simulink model "mediumFidelityScooterModel"  (R2022a)
settings: Solver=FixedStepAuto  StartTime=0  StopTime=50  FixedStep=Ts_mf  RelTol=1e-3  EnableMultiTasking=on
undefined symbols (not defined in the file): A, Cd, Crr, D, DiscIntNeverNeededParam, eff_gear, g, Ke, Kf, Ki_i, Ki_w, Kp_i, Kp_w, Kt, La, m_total, n_gear, Ra, rho, Rwheel, sigbuilder_block, slope, Tpeak, Vbat, Vnom
libraries: simulink x2, slpidlib x2
Description:
  | Medium fidelity simulation for control design validation
settings Model: Creator=The MathWorks, Inc.  LastModifiedBy=jdelolmo
settings SolverCC: AlgebraicLoopSolver=TrustRegion  AutoInsertRateTranBlk=on
settings DataIOCC: LimitDataPoints=on  ReturnWorkspaceOutputs=off
settings OptimizationCC: LifeSpan=inf
settings DebuggingCC: UnconnectedInputMsg=warning  UnconnectedOutputMsg=warning  UnconnectedLineMsg=warning  AllowSymbolicDim=off  SFUnexpectedBacktrackingDiag=warning  SFNoUnconditionalDefaultTransitionDiag=warning  SFExecutionAtInitializationDiag=none  SFMachineParentedDataDiag=warning  ArithmeticOperatorsInVariantConditions=warning
settings ModelReferenceCC: PropagateSignalLabelsOutOfModel=off
settings SFSimCC: SimUseLocalCustomCode=off  CustomCodeUndefinedFunction=UseInterfaceOnly
settings RTWCC: RTWUseLocalCustomCode=off  DLArmComputeVersion=19.05
settings CodeAppCC: StateflowObjectComments=on
settings GRTTargetCC: TargetLangStandard=C89/C90 (ANSI)
settings ConfigComp: CovMetricSettings=dw  CovSaveCumulativeToWorkspaceVar=on  CovSaveSingleToWorkspaceVar=on  CovExternalEMLEnable=off

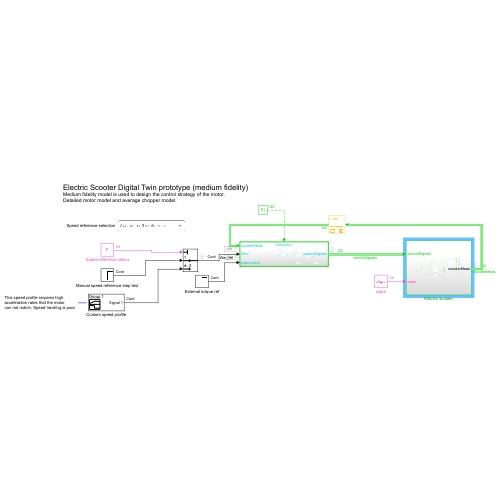
[thumbnail: Simulink's stored preview of the top-level diagram]
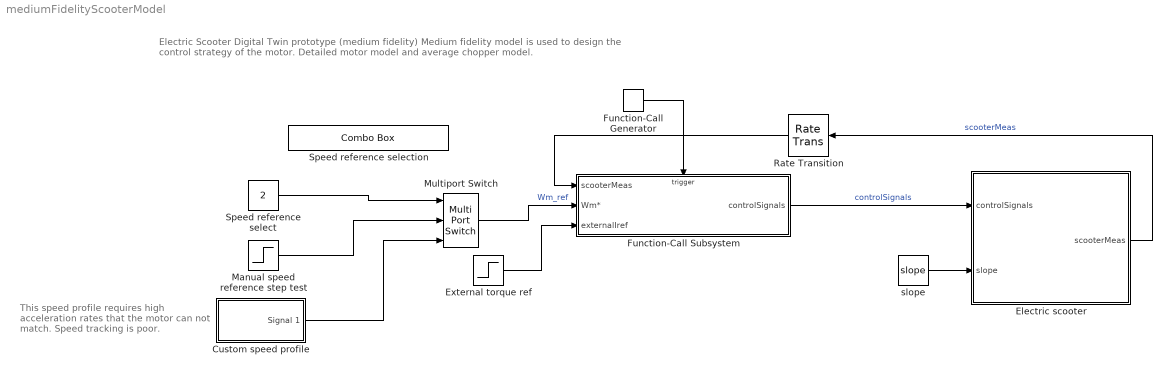
== system mediumFidelityScooterModel ==
  note: This speed profile requires high
      | acceleration rates that the motor
      | can not match. Speed tracking is poor.
  note: Electric Scooter Digital Twin prototype (medium fidelity)
      | Medium fidelity model is used to design the control strategy of the motor.
      | Detailed motor model and average chopper model.
  Custom speed profile : Subsystem  Tag=STV Subsys  LoadFcn=sigbuilder_block('load');  StartFcn=sigbuilder_block('start');  StopFcn=sigbuilder_block('stop');  ClipboardFcn=sigbuilder_block('clipboard');  mask(Sigbuilder block){tuvar=[0:10]}
      mask help: Simulink:masks:SigbuilderBlock_MD
      mask init:
      | if ~strcmp(get_param(bdroot(gcbh),'SimulationStatus'),'stopped') tuvar = sigbuilder_block('maskInit'); end
      settings: CopyFcn=sigbuilder_block('copy');  DeleteFcn=sigbuilder_block('delete');  ModelCloseFcn=sigbuilder_block('modelClose');  PreSaveFcn=sigbuilder_block('preSave');  PauseFcn=sigbuilder_block('pause');  ContinueFcn=sigbuilder_block('continue');  NameChangeFcn=sigbuilder_block('namechange');  OpenFcn=sigbuilder_block('open',[437.6 199.2 550.4 400 ]);  CloseFcn=sigbuilder_block('close');
      mask Display: plot(0, 0, 100, 100,[2, 2, 32, 32, 2], [68, 8, 8, 68, 68],[32, 2], [38, 38], [32, 19, 2],[53, 60, 44], [32, 17, 17, 2],[16, 16, 31, 31]);txt = getActiveGroup(gcbh);text(2, 100, txt,'verticalAlignment', 'top');
  Electric scooter : Subsystem
  External torque ref : Step  Time=0.1  After=Kt*16  SampleTime=0
  Function-Call Generator : simulink/Ports & Subsystems/Function-Call Generator  sample_time=Tcontrol  numberOfIterations=1  DisallowWideOutput=off
  Function-Call Subsystem : Subsystem  TreatAsAtomicUnit=on
  Manual speed reference step test : Step  Time=0.1  After=100  SampleTime=0
  Multiport Switch : MultiPortSwitch  Inputs=2  SaturateOnIntegerOverflow=off  InputSameDT=off
  Rate Transition : RateTransition  OutPortSampleTime=Tcontrol
  Speed reference select : Constant  Value=2
  Speed reference selection : ComboBox  LabelPosition=Hide  SelectedLabel=Custom profile reference
      settings: Values={{'Step reference', 'Custom profile reference', 'Vehicle profile'}, [1 2 3]}
  slope : Constant  Value=slope
  wires:
  Manual speed reference step test/1 -> Multiport Switch/2
  Speed reference select/1 -> Multiport Switch/1
  Custom speed profile/1(Signal 1) -> Multiport Switch/3
  slope/1 -> Electric scooter/2(slope)
  Function-Call Subsystem/1(controlSignals) -> Electric scooter/1(controlSignals)  "controlSignals"
  Function-Call Generator/1 -> Function-Call Subsystem/Trigger
  Electric scooter/1(scooterMeas) -> Rate Transition/1  "scooterMeas"
  Multiport Switch/1 -> Function-Call Subsystem/2(Wm*)  "Wm_ref"
  External torque ref/1 -> Function-Call Subsystem/3(externalIref)
  Rate Transition/1 -> Function-Call Subsystem/1(scooterMeas)

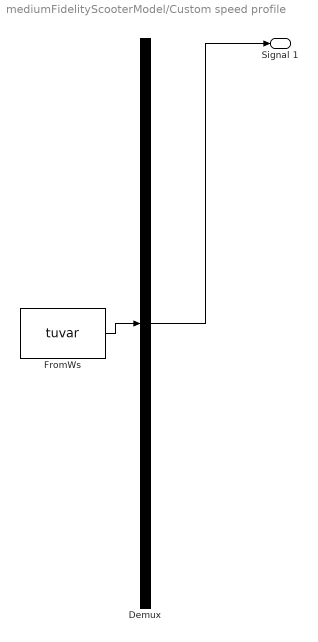
== system mediumFidelityScooterModel/Custom speed profile ==
  Demux : Demux  Tag=STV Demux  Outputs=1
      settings: DisplayOption=none
  FromWs : FromWorkspace  Tag=STV FromWs  VariableName=tuvar
      SigBuilderData=|
      | common.afterFinalStr = 'Extrapolate'
      | common.sampleTime = 0
      | dataSet.timeRange = [0 10]
      | dataSet.name = 'Group 1'
      | sbobj.Groups.Name = 'Group 1'
      | sbobj.Groups.Signals.Name = 'Signal 1'
      | sbobj.Groups.Signals.XData = [0 0.1 1.5 2 3 10]
      | sbobj.Groups.Signals.YData = [0 0 500 500 250 250]
  Signal 1 : Outport  Tag=STV Outport
  wires:
  Demux/1 -> Signal 1/1
  FromWs/1 -> Demux/1

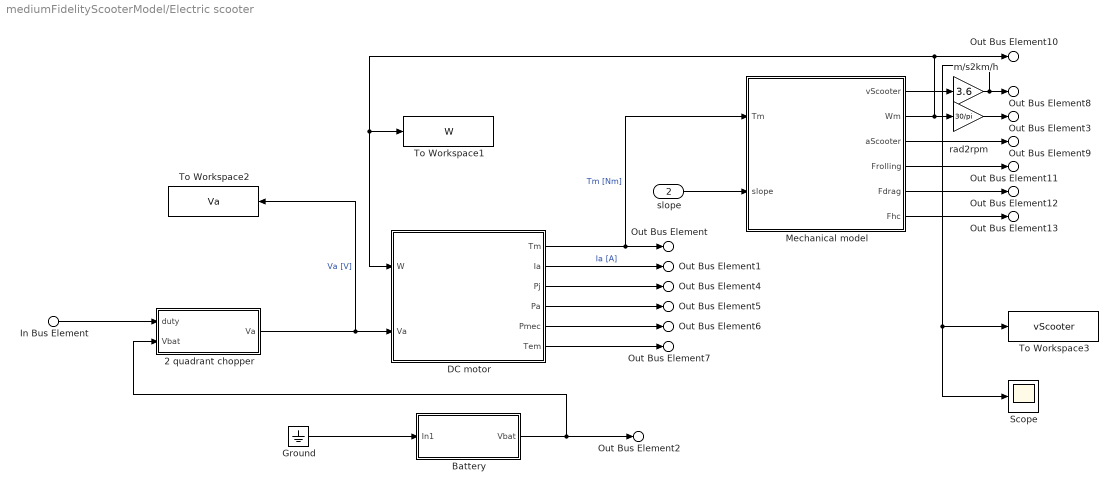
== system mediumFidelityScooterModel/Electric scooter ==
  In Bus Element : Inport  PortName=controlSignals  Element=duty
  slope : Inport  Port=2
  2 quadrant chopper : Subsystem
  Battery : Subsystem
  DC motor : Subsystem
  Ground : Ground
  Mechanical model : Subsystem
  Scope : Scope
  To Workspace1 : ToWorkspace  VariableName=W  SaveFormat=Timeseries  SampleTime=-1
  To Workspace2 : ToWorkspace  VariableName=Va  SaveFormat=Timeseries  SampleTime=-1
  To Workspace3 : ToWorkspace  VariableName=vScooter  SaveFormat=Timeseries  SampleTime=-1
  m/s2km/h : Gain  Gain=3.6
  rad2rpm : Gain  Gain=30/pi
  Out Bus Element : Outport  PortName=scooterMeas  Element=Tm
  Out Bus Element1 : Outport  PortName=scooterMeas  Element=Ia
  Out Bus Element2 : Outport  PortName=scooterMeas  Element=Vbat
  Out Bus Element4 : Outport  PortName=scooterMeas  Element=Pj
  Out Bus Element5 : Outport  PortName=scooterMeas  Element=Pa
  Out Bus Element6 : Outport  PortName=scooterMeas  Element=Pmec
  Out Bus Element7 : Outport  PortName=scooterMeas  Element=Tem
  Out Bus Element3 : Outport  PortName=scooterMeas  Element=WmRPM
  Out Bus Element8 : Outport  PortName=scooterMeas  Element=vScooter
  Out Bus Element9 : Outport  PortName=scooterMeas  Element=aScooter
  Out Bus Element10 : Outport  PortName=scooterMeas  Element=Wm
  Out Bus Element11 : Outport  PortName=scooterMeas  Element=Frolling
  Out Bus Element12 : Outport  PortName=scooterMeas  Element=Fdrag
  Out Bus Element13 : Outport  PortName=scooterMeas  Element=Fhc
  wires:
  DC motor/1(Tm) -> Mechanical model/1(Tm), Out Bus Element/1  "Tm [Nm]"
  DC motor/2(Ia) -> Out Bus Element1/1  "Ia [A]"
  Battery/1(Vbat) -> Out Bus Element2/1, 2 quadrant chopper/2(Vbat)
  Ground/1 -> Battery/1(In1)
  In Bus Element/1 -> 2 quadrant chopper/1(duty)
  2 quadrant chopper/1(Va) -> To Workspace2/1, DC motor/2(Va)  "Va [V]"
  DC motor/3(Pj) -> Out Bus Element4/1
  DC motor/4(Pa) -> Out Bus Element5/1
  DC motor/5(Pmec) -> Out Bus Element6/1
  DC motor/6(Tem) -> Out Bus Element7/1
  rad2rpm/1 -> Out Bus Element3/1
  Mechanical model/1(vScooter) -> m/s2km/h/1
  Mechanical model/2(Wm) -> rad2rpm/1, Out Bus Element10/1, To Workspace1/1, DC motor/1(W)
  Mechanical model/3(aScooter) -> Out Bus Element9/1
  slope/1 -> Mechanical model/2(slope)
  Mechanical model/4(Frolling) -> Out Bus Element11/1
  Mechanical model/5(Fdrag) -> Out Bus Element12/1
  Mechanical model/6(Fhc) -> Out Bus Element13/1
  m/s2km/h/1 -> Scope/1, To Workspace3/1, Out Bus Element8/1

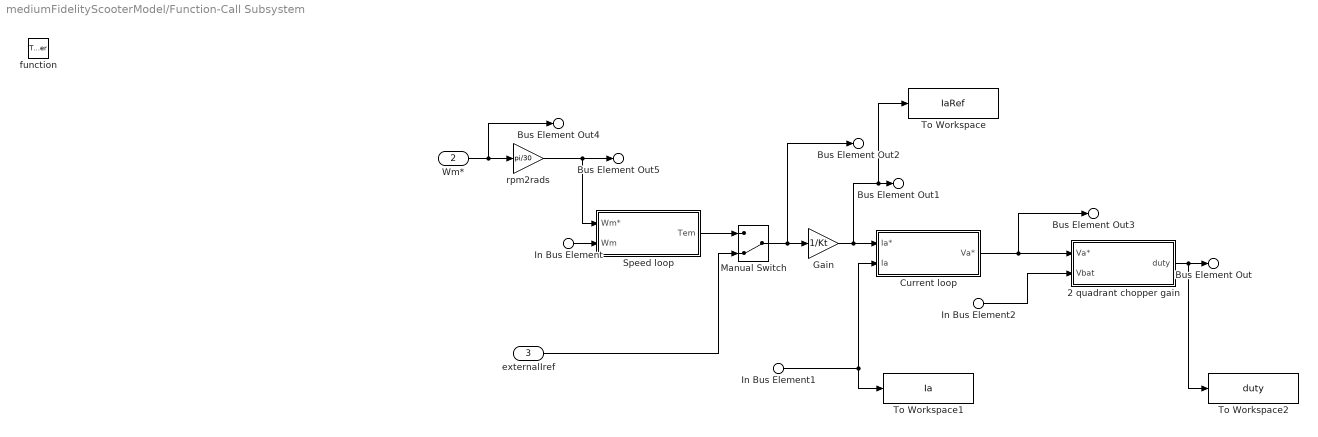
== system mediumFidelityScooterModel/Function-Call Subsystem ==
  In Bus Element1 : Inport  PortName=scooterMeas  Element=Ia
  In Bus Element : Inport  PortName=scooterMeas  Element=Wm
  In Bus Element2 : Inport  PortName=scooterMeas  Element=Vbat
  Wm* : Inport  Port=2
  externalIref : Inport  Port=3
  function : TriggerPort  TriggerType=function-call  VariantControl=(inherit)
  2 quadrant chopper gain : Subsystem
  Current loop : Subsystem
  Gain : Gain  Gain=1/Kt
  Manual Switch : ManualSwitch  CurrentSetting=0
  Speed loop : Subsystem
  To Workspace : ToWorkspace  VariableName=IaRef  SaveFormat=Timeseries  SampleTime=-1
  To Workspace1 : ToWorkspace  VariableName=Ia  SaveFormat=Timeseries  SampleTime=-1
  To Workspace2 : ToWorkspace  VariableName=duty  SaveFormat=Timeseries  SampleTime=-1
  rpm2rads : Gain  Gain=pi/30
  Bus Element Out : Outport  PortName=controlSignals  Element=duty
  Bus Element Out1 : Outport  PortName=controlSignals  Element=IaRef
  Bus Element Out2 : Outport  PortName=controlSignals  Element=TemRef
  Bus Element Out3 : Outport  PortName=controlSignals  Element=VaRef
  Bus Element Out4 : Outport  PortName=controlSignals  Element=WmRefRpm
  Bus Element Out5 : Outport  PortName=controlSignals  Element=WmRefRadS
  wires:
  externalIref/1 -> Manual Switch/2
  Wm*/1 -> Bus Element Out4/1, rpm2rads/1
  rpm2rads/1 -> Bus Element Out5/1, Speed loop/1(Wm*)
  Gain/1 -> To Workspace/1, Bus Element Out1/1, Current loop/1(Ia*)
  Speed loop/1(Tem) -> Manual Switch/1
  2 quadrant chopper gain/1(duty) -> To Workspace2/1, Bus Element Out/1
  In Bus Element/1 -> Speed loop/2(Wm)
  In Bus Element1/1 -> To Workspace1/1, Current loop/2(Ia)
  In Bus Element2/1 -> 2 quadrant chopper gain/2(Vbat)
  Current loop/1(Va*) -> Bus Element Out3/1, 2 quadrant chopper gain/1(Va*)
  Manual Switch/1 -> Bus Element Out2/1, Gain/1

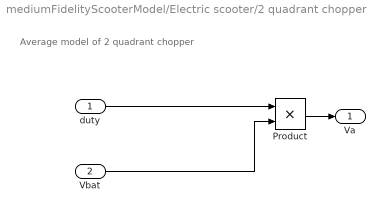
== system mediumFidelityScooterModel/Electric scooter/2 quadrant chopper ==
  note: Average model of 2 quadrant chopper
  duty : Inport
  Vbat : Inport  Port=2
  Product : Product
  Va : Outport
  wires:
  Vbat/1 -> Product/2
  duty/1 -> Product/1
  Product/1 -> Va/1

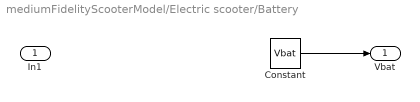
== system mediumFidelityScooterModel/Electric scooter/Battery ==
  In1 : Inport
  Constant : Constant  Value=Vbat
  Vbat : Outport
  wires:
  Constant/1 -> Vbat/1

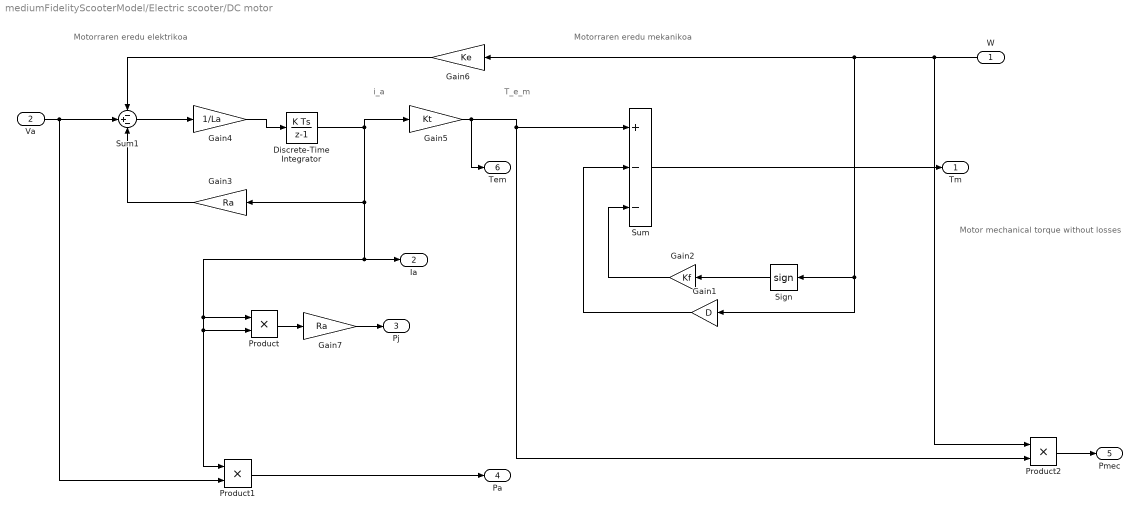
== system mediumFidelityScooterModel/Electric scooter/DC motor ==
  note: Motor mechanical torque without losses
  note: Motorraren eredu mekanikoa
  note: T_e_m
  note: Motorraren eredu elektrikoa
  note: i_a
  W : Inport
  Va : Inport  Port=2
  Discrete-Time Integrator : DiscreteIntegrator  SampleTime=200e-6  ICPrevOutput=DiscIntNeverNeededParam  ICPrevScaledInput=DiscIntNeverNeededParam
  Gain1 : Gain  Gain=D
  Gain2 : Gain  Gain=Kf
  Gain3 : Gain  Gain=Ra
  Gain4 : Gain  Gain=1/La
  Gain5 : Gain  Gain=Kt
  Gain6 : Gain  Gain=Ke
  Gain7 : Gain  Gain=Ra
  Product : Product
  Product1 : Product
  Product2 : Product
  Sign : Signum
  Sum : Sum  Inputs=+--
  Sum1 : Sum  Inputs=-+-
  Tm : Outport  VectorParamsAs1DForOutWhenUnconnected=off
  Ia : Outport  Port=2  VectorParamsAs1DForOutWhenUnconnected=off
  Pj : Outport  Port=3  VectorParamsAs1DForOutWhenUnconnected=off
  Pa : Outport  Port=4  VectorParamsAs1DForOutWhenUnconnected=off
  Pmec : Outport  Port=5  VectorParamsAs1DForOutWhenUnconnected=off
  Tem : Outport  Port=6  VectorParamsAs1DForOutWhenUnconnected=off
  wires:
  Gain4/1 -> Discrete-Time Integrator/1
  Sum1/1 -> Gain4/1
  Sign/1 -> Gain2/1
  Gain3/1 -> Sum1/3
  Gain1/1 -> Sum/2
  Va/1 -> Product1/2, Sum1/2
  Gain5/1 -> Tem/1, Sum/1, Product2/2
  Sum/1 -> Tm/1
  Discrete-Time Integrator/1 -> Gain5/1, Product/1, Product/2, Product1/1, Ia/1, Gain3/1
  Gain6/1 -> Sum1/1
  Gain7/1 -> Pj/1
  Product/1 -> Gain7/1
  Product1/1 -> Pa/1
  Product2/1 -> Pmec/1
  Gain2/1 -> Sum/3
  W/1 -> Product2/1, Gain1/1, Sign/1, Gain6/1

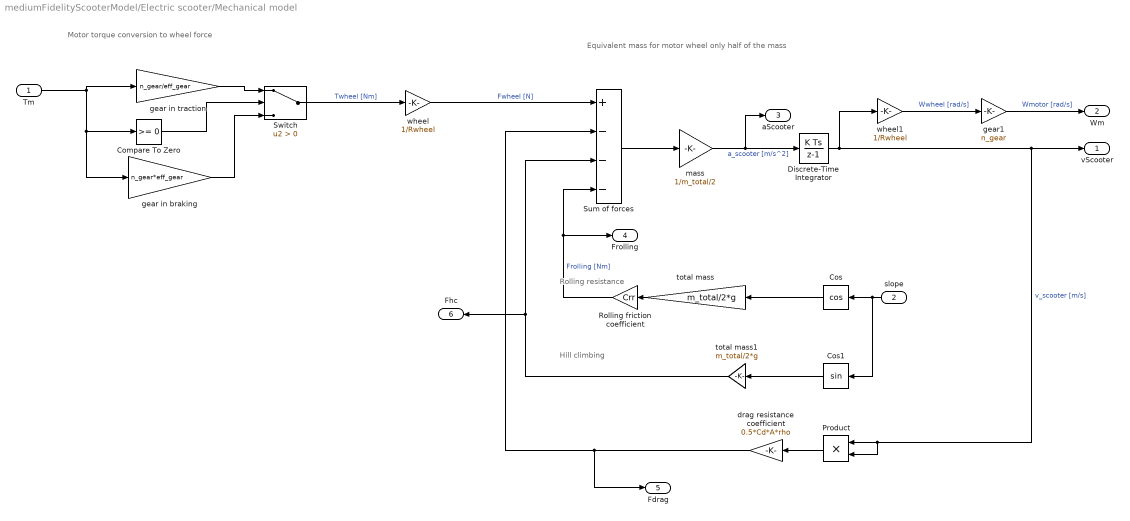
== system mediumFidelityScooterModel/Electric scooter/Mechanical model ==
  note: Hill climbing
  note: Motor torque conversion to wheel force
  note: Equivalent mass for motor wheel only half of the mass
  note: Rolling resistance
  Tm : Inport
  slope : Inport  Port=2
  Compare To Zero : simulink/Logic and Bit Operations/Compare To Zero  relop=>=  OutDataTypeStr=boolean
  Cos : Trigonometry  Operator=cos
  Cos1 : Trigonometry
  Discrete-Time Integrator : DiscreteIntegrator  SampleTime=200e-6  ICPrevOutput=DiscIntNeverNeededParam  ICPrevScaledInput=DiscIntNeverNeededParam
  Product : Product
  Rolling friction coefficient : Gain  Gain=Crr
  Sum of forces : Sum  Inputs=+---
  Switch : Switch  Criteria=u2 > Threshold  SaturateOnIntegerOverflow=off  InputSameDT=off
  drag resistance coefficient : Gain  Gain=0.5*Cd*A*rho
  gear in braking : Gain  Gain=n_gear*eff_gear
  gear in traction : Gain  Gain=n_gear/eff_gear
  gear1 : Gain  Gain=n_gear
  mass : Gain  Gain=1/m_total/2
  total mass : Gain  Gain=m_total/2*g
  total mass1 : Gain  Gain=m_total/2*g
  wheel : Gain  Gain=1/Rwheel
  wheel1 : Gain  Gain=1/Rwheel
  vScooter : Outport
  Wm : Outport  Port=2
  aScooter : Outport  Port=3
  Frolling : Outport  Port=4
  Fdrag : Outport  Port=5
  Fhc : Outport  Port=6
  wires:
  Tm/1 -> Compare To Zero/1, gear in braking/1, gear in traction/1
  wheel/1 -> Sum of forces/1  "Fwheel [N]"
  Sum of forces/1 -> mass/1
  mass/1 -> Discrete-Time Integrator/1, aScooter/1  "a_scooter [m/s^2]"
  Discrete-Time Integrator/1 -> Product/2, Product/1, vScooter/1, wheel1/1  "v_scooter [m/s]"
  wheel1/1 -> gear1/1  "Wwheel [rad/s]"
  gear1/1 -> Wm/1  "Wmotor [rad/s]"
  Switch/1 -> wheel/1  "Twheel [Nm]"
  gear in traction/1 -> Switch/1
  gear in braking/1 -> Switch/3
  Compare To Zero/1 -> Switch/2
  Rolling friction coefficient/1 -> Frolling/1, Sum of forces/4  "Frolling [Nm]"
  total mass/1 -> Rolling friction coefficient/1
  Cos/1 -> total mass/1
  slope/1 -> Cos1/1, Cos/1
  Cos1/1 -> total mass1/1
  total mass1/1 -> Fhc/1, Sum of forces/3
  Product/1 -> drag resistance coefficient/1
  drag resistance coefficient/1 -> Fdrag/1, Sum of forces/2

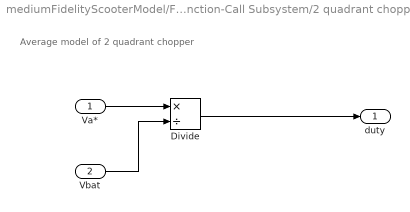
== system mediumFidelityScooterModel/Function-Call Subsystem/2 quadrant chopper gain ==
  note: Average model of 2 quadrant chopper
  Va* : Inport
  Vbat : Inport  Port=2
  Divide : Product  Inputs=*/
  duty : Outport
  wires:
  Divide/1 -> duty/1
  Va*/1 -> Divide/1
  Vbat/1 -> Divide/2

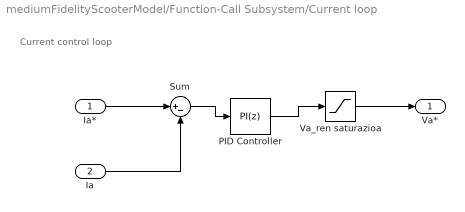
== system mediumFidelityScooterModel/Function-Call Subsystem/Current loop ==
  note: Current control loop
  Ia* : Inport
  Ia : Inport  Port=2
  PID Controller : slpidlib/PID Controller  Controller=PI  Form=Parallel  TimeDomain=Discrete-time  UseExternalTs=off  SampleTime=-1  IntegratorMethod=Forward Euler  FilterMethod=Forward Euler  ControllerParametersSource=internal  P=Kp_i  I=Ki_i  UseKiTs=off  D=0  N=100  UseFilter=on  TunerSelectOption=Transfer Function Based (PID Tuner App)  InitialConditionSource=internal  InitialConditionForIntegrator=0  InitialConditionForFilter=0  DifferentiatorICPrevScaledInput=0  ExternalReset=none  TrackingMode=off  Kt=1  LimitOutput=on  SatLimitsSource=internal  UpperSaturationLimit=inf  LowerSaturationLimit=-inf  LinearizeAsGain=on  AntiWindupMode=back-calculation  Kb=1  POutMin=[]  POutMax=[]  IOutMin=[]  IOutMax=[]  DOutMin=[]  DOutMax=[]  NOutMin=[]  NOutMax=[]  SumOutMin=[]  SumOutMax=[]  SaturationOutMin=[]  SaturationOutMax=[]  PParamMin=[]  PParamMax=[]  IParamMin=[]  IParamMax=[]  DParamMin=[]  DParamMax=[]  NParamMin=[]  NParamMax=[]  KbParamMin=[]  KbParamMax=[]  KtParamMin=[]  KtParamMax=[]  KbOutMin=[]  KbOutMax=[]  KtOutMin=[]  KtOutMax=[]  IntegratorOutMin=[]  IntegratorOutMax=[]  FilterOutMin=[]  FilterOutMax=[]  SumI1OutMin=[]  SumI1OutMax=[]  SumI2OutMin=[]  SumI2OutMax=[]  SumI3OutMin=[]  SumI3OutMax=[]  SumI4OutMin=[]  SumI4OutMax=[]  SumDOutMin=[]  SumDOutMax=[]  DifferentiatorOutMin=[]  DifferentiatorOutMax=[]  FilterDiffOutCoefMin=[]  FilterDiffOutCoefMax=[]  ReciprocalOutMin=[]  ReciprocalOutMax=[]  SumDenOutMin=[]  SumDenOutMax=[]  SumNumOutMin=[]  SumNumOutMax=[]  DivideOutMin=[]  DivideOutMax=[]  UdiffTsProdOutMin=[]  UdiffTsProdOutMax=[]  NTsProdOutMin=[]  NTsProdOutMax=[]  UintegralTsProdOutMin=[]  UintegralTsProdOutMax=[]  UngainTsProdOutMin=[]  UngainTsProdOutMax=[]  IntegratorContinuousStateAttributes=''  IntegratorStateMustResolveToSignalObject=off  IntegratorRTWStateStorageClass=Auto  FilterContinuousStateAttributes=''  FilterStateMustResolveToSignalObject=off  FilterRTWStateStorageClass=Auto  ParallelPVariant=InternalParameters  IdealPVariant=Disabled  IVariant=InternalParameters  DVariant=Disabled  IntegratorVariant=Discrete  SatVariant=Enabled  AWVariant=BackCalculation  PCopyVariant=Disabled  TRVariant=Disabled  FdbkBlocksVariant=Forward  IdealPFdbkVariant=Disabled  SatFdbkVariant=Disabled  DerivativeFilterVariant=Disabled  NVariant=Disabled  NCopyVariant=Disabled_SignalSpec  FilterICVariant=Disabled  IntegratorICVariant=InternalICs  ExternalResetVariant=Disabled  TRSumVariant=Passthrough  SumFdbkVariant=Disabled  SumVariant=Sum_PI  TsampFilterVariant=InternalTs  TsampNgainVariant=Passthrough  TsampIntegralVariant=Passthrough  ExternalSaturationOutDataTypeStr=Inherit: Same as second input  aMode=0
  Sum : Sum  Inputs=|+-
  Va_ren saturazioa : Saturate  UpperLimit=Vnom  LowerLimit=0
  Va* : Outport
  wires:
  Ia/1 -> Sum/2
  Ia*/1 -> Sum/1
  Sum/1 -> PID Controller/1
  PID Controller/1 -> Va_ren saturazioa/1
  Va_ren saturazioa/1 -> Va*/1

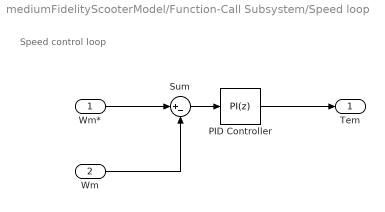
== system mediumFidelityScooterModel/Function-Call Subsystem/Speed loop ==
  note: Speed control loop
  Wm* : Inport
  Wm : Inport  Port=2
  PID Controller : slpidlib/PID Controller  Controller=PI  Form=Parallel  TimeDomain=Discrete-time  UseExternalTs=off  SampleTime=-1  IntegratorMethod=Forward Euler  FilterMethod=Forward Euler  ControllerParametersSource=internal  P=Kp_w  I=Ki_w  UseKiTs=off  D=0  N=100  UseFilter=on  TunerSelectOption=Transfer Function Based (PID Tuner App)  InitialConditionSource=internal  InitialConditionForIntegrator=0  InitialConditionForFilter=0  DifferentiatorICPrevScaledInput=0  ExternalReset=none  TrackingMode=off  Kt=1  LimitOutput=on  SatLimitsSource=internal  UpperSaturationLimit=Tpeak  LowerSaturationLimit=-Tpeak  LinearizeAsGain=on  AntiWindupMode=clamping  Kb=1  POutMin=[]  POutMax=[]  IOutMin=[]  IOutMax=[]  DOutMin=[]  DOutMax=[]  NOutMin=[]  NOutMax=[]  SumOutMin=[]  SumOutMax=[]  SaturationOutMin=[]  SaturationOutMax=[]  PParamMin=[]  PParamMax=[]  IParamMin=[]  IParamMax=[]  DParamMin=[]  DParamMax=[]  NParamMin=[]  NParamMax=[]  KbParamMin=[]  KbParamMax=[]  KtParamMin=[]  KtParamMax=[]  KbOutMin=[]  KbOutMax=[]  KtOutMin=[]  KtOutMax=[]  IntegratorOutMin=[]  IntegratorOutMax=[]  FilterOutMin=[]  FilterOutMax=[]  SumI1OutMin=[]  SumI1OutMax=[]  SumI2OutMin=[]  SumI2OutMax=[]  SumI3OutMin=[]  SumI3OutMax=[]  SumI4OutMin=[]  SumI4OutMax=[]  SumDOutMin=[]  SumDOutMax=[]  DifferentiatorOutMin=[]  DifferentiatorOutMax=[]  FilterDiffOutCoefMin=[]  FilterDiffOutCoefMax=[]  ReciprocalOutMin=[]  ReciprocalOutMax=[]  SumDenOutMin=[]  SumDenOutMax=[]  SumNumOutMin=[]  SumNumOutMax=[]  DivideOutMin=[]  DivideOutMax=[]  UdiffTsProdOutMin=[]  UdiffTsProdOutMax=[]  NTsProdOutMin=[]  NTsProdOutMax=[]  UintegralTsProdOutMin=[]  UintegralTsProdOutMax=[]  UngainTsProdOutMin=[]  UngainTsProdOutMax=[]  IntegratorContinuousStateAttributes=''  IntegratorStateMustResolveToSignalObject=off  IntegratorRTWStateStorageClass=Auto  FilterContinuousStateAttributes=''  FilterStateMustResolveToSignalObject=off  FilterRTWStateStorageClass=Auto  ParallelPVariant=InternalParameters  IdealPVariant=Disabled  IVariant=InternalParameters  DVariant=Disabled  IntegratorVariant=Discrete  SatVariant=Enabled  AWVariant=DiscClampingParallel  PCopyVariant=Disabled  TRVariant=Disabled  FdbkBlocksVariant=Forward  IdealPFdbkVariant=Disabled  SatFdbkVariant=Disabled  DerivativeFilterVariant=Disabled  NVariant=Disabled  NCopyVariant=Disabled_SignalSpec  FilterICVariant=Disabled  IntegratorICVariant=InternalICs  ExternalResetVariant=Disabled  TRSumVariant=Passthrough  SumFdbkVariant=Disabled  SumVariant=Sum_PI  TsampFilterVariant=InternalTs  TsampNgainVariant=Passthrough  TsampIntegralVariant=Passthrough  ExternalSaturationOutDataTypeStr=Inherit: Same as second input  aMode=0
  Sum : Sum  Inputs=|+-
  Tem : Outport
  wires:
  PID Controller/1 -> Tem/1
  Sum/1 -> PID Controller/1
  Wm*/1 -> Sum/1
  Wm/1 -> Sum/2
